simulink subsystem "state"  (R2019b)
settings: Solver=VariableStepAuto  StartTime=0.0  StopTime=10.0  RelTol=1e-3
InitFcn:
  | %% DSPBuilder Start
  | alt_dspbuilder_update_model(bdroot)
  | %% DSPBuilder End
StartFcn:
  | %% DSPBuilder Start
  | alt_dspbuilder_hdlimport_prepare_for_simulation(bdroot)
  | %% DSPBuilder End
libraries: allblocks_alteradspbuilder2 x5
settings Model: Creator=vboxuser  LastModifiedBy=vboxuser

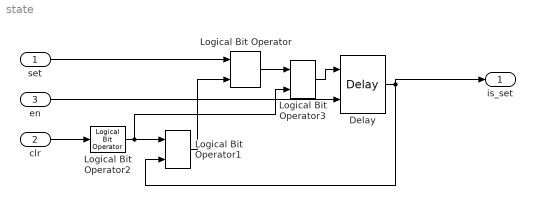
== system state ==
  set : Inport
  clr : Inport  Port=2
  en : Inport  Port=3
  Delay : allblocks_alteradspbuilder2/Delay  pipeline=1  pipeline_display=1  ClockPhase=1  use_ena=on  use_sclr=off  allowFloatingPointOverride=on  logOutputs=off  logFile=C:\Users\vboxuser\Documents\MATLAB\serializer\tb_sync_simu\sync%5Fsimu_Subsystem+Reference1_NOT%5FMATCHING_Delay.fixedpointlog  use_init=off  reset_value=1
  Logical Bit Operator : allblocks_alteradspbuilder2/Logical Bit Operator  LogicalOperator=OR  user_inputs=2  pipeline_display=0
  Logical Bit Operator1 : allblocks_alteradspbuilder2/Logical Bit Operator  LogicalOperator=AND  user_inputs=2  pipeline_display=0
  Logical Bit Operator2 : allblocks_alteradspbuilder2/Logical Bit Operator  LogicalOperator=NOT  user_inputs=2  pipeline_display=0
  Logical Bit Operator3 : allblocks_alteradspbuilder2/Logical Bit Operator  LogicalOperator=AND  user_inputs=2  pipeline_display=0
  is_set : Outport
  wires:
  en/1 -> Delay/2
  Logical Bit Operator1/1 -> Logical Bit Operator/2
  Delay/1 -> is_set/1, Logical Bit Operator1/2
  clr/1 -> Logical Bit Operator2/1
  set/1 -> Logical Bit Operator/1
  Logical Bit Operator/1 -> Logical Bit Operator3/1
  Logical Bit Operator2/1 -> Logical Bit Operator1/1, Logical Bit Operator3/2
  Logical Bit Operator3/1 -> Delay/1
